simulink model "Hybrid_Series"  (R2017b)
settings: Solver=VariableStepAuto  StartTime=0.0  StopTime=20  RelTol=1e-3  AbsTol=1e-3  EnableMultiTasking=on
model workspace (MATLAB code in the model file):
  | v0                 = 15; % Initial vehicle speed
  | wheel_radius = 0.3; % Wheel radius
  | k                   = 1e-2; % Motor losses (W/(N*M)^2)
  | t_torque        = 0.02; % Electric motor time constant
  | rpm0             = 2000; % Engine initial speed demand
values from neighbouring files (symbols this model uses):
  HEV_Param =     [DataWorkSpace.mat]
libraries: fl_lib x83, nesl_utility x27, sdl_lib x5, elec_lib x2
(part 2 of 2)

== system Hybrid_Series/DC Converter/Thermal Model ==
  Air Temperature : fl_lib/Physical Signals/Sources/PS Constant  constant=HEV_Param.DCDCConv.Air_Temperature
  Ideal Heat Flow Source : fl_lib/Thermal/Thermal Sources/Controlled Heat Flow Rate Source
      settings: SourceProductName=Simscape
  Ideal Temperature Source : fl_lib/Thermal/Thermal Sources/Controlled Temperature Source
      settings: SourceProductName=Simscape
  Nominal Case-Atmosphere Convective Heat Transfer : fl_lib/Thermal/Thermal Elements/Convective Heat Transfer  area=HEV_Param.DCDCConv.Convection.Area cm^2  heat_tr_coeff=HEV_Param.DCDCConv.Convection.HT_Coefficient W/(m^2 *K)  T_specify=off  T_priority=High  T=0 K  T_nominal_specify=off  T_nominal_unit=K  T_nominal_value=1  Q_specify=off  Q_priority=High  Q=0 J/s  Q_nominal_specify=off  Q_nominal_unit=J/s  Q_nominal_value=1
  PtoHeat : fl_lib/Physical Signals/Functions/PS Gain  gain=HEV_Param.DCDCConv.EPower2Heat
  Subsystem : Subsystem
      mask Display: disp('S');
  Temperature Sensor : Subsystem
      mask Display:
      | patch([294.730220921338;294.546109275896;293.995547435362;293.083837611228;291.819760067491;290.215488561913;288.286473106077;286.051291173329;283.531468787557;280.75127321581;277.737479261253;274.519111407178;271.127164295357;267.594304230703;263.954554586898;260.242968142701;256.495289504528;252.747610866356;249.036024422158;245.396274778353;241.8634147137;238.471467601878;235.253099747803;232.239305793246;229.459110221499;226.939287835727;224.704105902979;222.775090447143;221.170818941565;219.906741397828;218.995031573694;218.44446973316;218.260358087718;218.44446973316;218.995031573694;219.906741397828;221.170818941565;222.775090447143;224.704105902979;226.939287835727;229.459110221499;232.239305793247;235.253099747803;238.471467601878;241.8634147137;245.396274778353;249.036024422158;252.747610866356;256.495289504528;260.242968142701;263.954554586898;267.594304230703;271.127164295357;274.519111407178;277.737479261253;280.75127321581;283.531468787557;286.051291173329;288.286473106077;290.215488561913;291.819760067491;293.083837611228;293.995547435362;294.546109275896;294.730220921338;294.730220921338], [122.389574535191;118.641895897019;114.930309452821;111.290559809016;107.757699744363;104.365752632541;101.147384778466;98.1335908239095;95.3533952521624;92.8335728663899;90.598390933642;88.6693754778057;87.0651039722279;85.8010264284914;84.8893166043572;84.3387547638233;84.1546431183815;84.3387547638233;84.8893166043572;85.8010264284914;87.0651039722279;88.6693754778058;90.598390933642;92.83357286639;95.3533952521625;98.1335908239095;101.147384778466;104.365752632541;107.757699744363;111.290559809016;114.930309452821;118.641895897019;122.389574535191;126.137253173364;129.848839617561;133.488589261366;137.02144932602;140.413396437841;143.631764291917;146.645558246473;149.42575381822;151.945576203992;154.18075813674;156.109773592576;157.714045098154;158.978122641891;159.889832466025;160.440394306559;160.624505952001;160.440394306559;159.889832466025;158.978122641891;157.714045098154;156.109773592576;154.18075813674;151.945576203992;149.42575381822;146.645558246473;143.631764291917;140.413396437841;137.02144932602;133.488589261366;129.848839617561;126.137253173364;122.389574535191;122.389574535191], [0;0;0])
      | plot([294.730220921338;294.546109275896;293.995547435362;293.083837611228;291.819760067491;290.215488561913;288.286473106077;286.051291173329;283.531468787557;280.75127321581;277.737479261253;274.519111407178;271.127164295357;267.594304230703;263.954554586898;260.242968142701;256.495289504528;252.747610866356;249.036024422158;245.396274778353;241.8634147137;238.471467601878;235.253099747803;232.239305793246;229.459110221499;226.939287835727;224.704105902979;222.775090447143;221.170818941565;219.906741397828;218.995031573694;218.44446973316;218.260358087718;218.44446973316;218.995031573694;219.906741397828;221.170818941565;222.775090447143;224.704105902979;226.939287835727;229.459110221499;232.239305793247;235.253099747803;238.471467601878;241.8634147137;245.396274778353;249.036024422158;252.747610866356;256.495289504528;260.242968142701;263.954554586898;267.594304230703;271.127164295357;274.519111407178;277.737479261253;280.75127321581;283.531468787557;286.051291173329;288.286473106077;290.215488561913;291.819760067491;293.083837611228;293.995547435362;294.546109275896;294.730220921338;294.730220921338], [122.389574535191;118.641895897019;114.930309452821;111.290559809016;107.757699744363;104.365752632541;101.147384778466;98.1335908239095;95.3533952521624;92.8335728663899;90.598390933642;88.6693754778057;87.0651039722279;85.8010264284914;84.8893166043572;84.3387547638233;84.1546431183815;84.3387547638233;84.8893166043572;85.8010264284914;87.0651039722279;88.6693754778058;90.598390933642;92.83357286639;95.3533952521625;98.1335908239095;101.147384778466;104.365752632541;107.757699744363;111.290559809016;114.930309452821;118.641895897019;122.389574535191;126.137253173364;129.848839617561;133.488589261366;137.02144932602;140.413396437841;143.631764291917;146.645558246473;149.42575381822;151.945576203992;154.18075813674;156.109773592576;157.714045098154;158.978122641891;159.889832466025;160.440394306559;160.624505952001;160.440394306559;159.889832466025;158.978122641891;157.714045098154;156.109773592576;154.18075813674;151.945576203992;149.42575381822;146.645558246473;143.631764291917;140.413396437841;137.02144932602;133.488589261366;129.848839617561;126.137253173364;122.389574535191;122.389574535191])
      | plot([243.771309033036;263.613159768283;263.613159768283;243.771309033036;243.771309033036], [438.410416245461;438.410416245461;112.4371541664;112.4371541664;438.410416245461])
      | plot([510.219018906355;0;0;510.219018906355;510.219018906355], [509.274168871343;509.274168871343;0;0;509.274168871343])
      | ;
      | %color('red');
      | %port_label('LConn', 1,'A')
      | %port_label('RConn', 1,'B')
  Thermal Mass : fl_lib/Thermal/Thermal Elements/Thermal Mass  mass=HEV_Param.DCDCConv.Thermal_Mass kg  sp_heat=HEV_Param.DCDCConv.Specific_Heat J/kg/K  T_specify=on  T_priority=High  T=HEV_Param.DCDCConv.Initial_Temperature degC  T_nominal_specify=off  T_nominal_unit=K  T_nominal_value=1  Q_specify=off  Q_priority=High  Q=0 J/s  Q_nominal_specify=off  Q_nominal_unit=J/s  Q_nominal_value=1
  Thermal Reference : fl_lib/Thermal/Thermal Elements/Thermal Reference
  Thermal Reference1 : fl_lib/Thermal/Thermal Elements/Thermal Reference
  P Loss : PMIOPort  Port=1  Side=Left
  connections:
  Thermal Reference1/LConn1 -- Ideal Heat Flow Source/RConn2
  PtoHeat/LConn1 -- Subsystem/RConn1
  Subsystem/LConn1 -- P Loss/RConn1
  Air Temperature/RConn1 -- Ideal Temperature Source/RConn1
  Ideal Temperature Source/RConn2 -- Thermal Reference/LConn1
  PtoHeat/RConn1 -- Ideal Heat Flow Source/RConn1
  Ideal Heat Flow Source/LConn1 -- Thermal Mass/LConn1 -- Nominal Case-Atmosphere Convective Heat Transfer/RConn1 -- Temperature Sensor/LConn1
  Nominal Case-Atmosphere Convective Heat Transfer/LConn1 -- Ideal Temperature Source/LConn1

== system Hybrid_Series/DC Converter/Voltage Sensor ==
  PS-Simulink Converter : nesl_utility/PS-Simulink Converter  PhysicalDomain=network_engine_domain  SubClassName=ps_output  LeftPortType=input  RightPortType=output  PseudoPeriodic=off  Frequencies=[]  Unit=1  AffineConversion=off
  Voltage Sensor In : fl_lib/Electrical/Electrical Sensors/Voltage Sensor
  + : PMIOPort  Port=1  Side=Left
  V : PMIOPort  Port=2  Side=Right
  - : PMIOPort  Port=3  Side=Right
  tag scope: V_in=global
  wires:
  PS-Simulink Converter/1 -> [V_in]
  connections:
  PS-Simulink Converter/LConn1 -- Voltage Sensor In/RConn1 -- V/RConn1
  -/RConn1 -- Voltage Sensor In/RConn2
  +/RConn1 -- Voltage Sensor In/LConn1

== system Hybrid_Series/DC Converter/Voltage Sensor Bus ==
  PS-Simulink Converter : nesl_utility/PS-Simulink Converter  PhysicalDomain=network_engine_domain  SubClassName=ps_output  LeftPortType=input  RightPortType=output  PseudoPeriodic=off  Frequencies=[]  Unit=1  AffineConversion=off
  Voltage Sensor Out : fl_lib/Electrical/Electrical Sensors/Voltage Sensor
  + : PMIOPort  Port=1  Side=Left
  - : PMIOPort  Port=2  Side=Right
  V : PMIOPort  Port=3  Side=Right
  tag scope: V_out=global
  wires:
  PS-Simulink Converter/1 -> [V_out]
  connections:
  -/RConn1 -- Voltage Sensor Out/RConn2
  PS-Simulink Converter/LConn1 -- Voltage Sensor Out/RConn1 -- V/RConn1
  +/RConn1 -- Voltage Sensor Out/LConn1

== system Hybrid_Series/Engine/Engine Management ==
  rpm_dem : Inport
  rpm : Inport  Port=2
  Kp : Gain  Gain=1e-3  SaturateOnIntegerOverflow=on  OutDataTypeStr=Inherit: Same as input  ParamDataTypeStr=Inherit: Same as input
  Sum2 : Sum  Inputs=+-|  SaturateOnIntegerOverflow=on  InputSameDT=on  OutDataTypeStr=Inherit: Same as first input
  "[0,1]" : Saturate  UpperLimit=1  LowerLimit=0
  T : Outport
  wires:
  rpm/1 -> Sum2/2
  rpm_dem/1 -> Sum2/1
  Sum2/1 -> Kp/1
  Kp/1 -> "[0,1]"/1
  "[0,1]"/1 -> T/1

== system Hybrid_Series/Engine/RPM Sensor ==
  Ideal Rotational Motion Sensor : fl_lib/Mechanical/Mechanical Sensors/Ideal Rotational Motion Sensor  offset=0 rad
  MRR : fl_lib/Mechanical/Rotational Elements/Mechanical Rotational Reference
  PS2S : nesl_utility/PS-Simulink Converter  PhysicalDomain=network_engine_domain  SubClassName=ps_output  LeftPortType=input  RightPortType=output  PseudoPeriodic=off  Frequencies=[]  Unit=rpm  AffineConversion=off
  Sensor dynamics : TransferFcn  Denominator=[0.01 1]
  F : PMIOPort  Port=1  Side=Left
  rpm : Outport
  tag scope: engine_rpm=global
  wires:
  PS2S/1 -> Sensor dynamics/1, [engine_rpm]
  Sensor dynamics/1 -> rpm/1
  connections:
  F/RConn1 -- Ideal Rotational Motion Sensor/LConn1
  Ideal Rotational Motion Sensor/RConn2 -- PS2S/LConn1
  MRR/LConn1 -- Ideal Rotational Motion Sensor/RConn1

== system Hybrid_Series/Engine/Sensor Fuel ==
  Integrator : Integrator
  PS2S2 : nesl_utility/PS-Simulink Converter  PhysicalDomain=network_engine_domain  SubClassName=ps_output  LeftPortType=input  RightPortType=output  PseudoPeriodic=off  Frequencies=[]  Unit=g/s  AffineConversion=off
  FC : PMIOPort  Port=1  Side=Left
  tag scope: Fuel=global
  wires:
  PS2S2/1 -> Integrator/1
  Integrator/1 -> [Fuel]
  connections:
  FC/RConn1 -- PS2S2/LConn1

== system Hybrid_Series/Engine/Sensor Power ==
  PS2S1 : nesl_utility/PS-Simulink Converter  PhysicalDomain=network_engine_domain  SubClassName=ps_output  LeftPortType=input  RightPortType=output  PseudoPeriodic=off  Frequencies=[]  Unit=kW  AffineConversion=off
  P : PMIOPort  Port=1  Side=Left
  tag scope: Pm_engine=global
  wires:
  PS2S1/1 -> [Pm_engine]
  connections:
  P/RConn1 -- PS2S1/LConn1

== system Hybrid_Series/Generator/Power Sensor ==
  Current Sensor : fl_lib/Electrical/Electrical Sensors/Current Sensor
  PS Product1 : fl_lib/Physical Signals/Functions/PS Product
      settings: SourceProductName=Simscape
  PS-Simulink Converter4 : nesl_utility/PS-Simulink Converter  PhysicalDomain=network_engine_domain  SubClassName=ps_output  LeftPortType=input  RightPortType=output  PseudoPeriodic=off  Frequencies=[]  Unit=N*m  AffineConversion=off
  To Workspace : ToWorkspace  VariableName=powerGen  SampleTime=-1
      settings: Save2DSignal=2-D array (concatenate along first dimension)
  Voltage Sensor : fl_lib/Electrical/Electrical Sensors/Voltage Sensor
  W to kW : Gain  Gain=1/1000
  + : PMIOPort  Port=1  Side=Left
  ref : PMIOPort  Port=2  Side=Left
  - : PMIOPort  Port=3  Side=Right
  tag scope: Pe_gen=global
  wires:
  W to kW/1 -> To Workspace/1, [Pe_gen]
  PS-Simulink Converter4/1 -> W to kW/1
  connections:
  Current Sensor/RConn1 -- PS Product1/LConn1
  -/RConn1 -- Current Sensor/RConn2 -- Voltage Sensor/LConn1
  Voltage Sensor/RConn1 -- PS Product1/LConn2
  PS-Simulink Converter4/LConn1 -- PS Product1/RConn1
  +/RConn1 -- Current Sensor/LConn1
  ref/RConn1 -- Voltage Sensor/RConn2

== system Hybrid_Series/Generator/RPM Sensor ==
  Mechanical Rotational Reference : fl_lib/Mechanical/Rotational Elements/Mechanical Rotational Reference
  Motion Sensor : fl_lib/Mechanical/Mechanical Sensors/Ideal Rotational Motion Sensor  offset=0 rad
  PS-Simulink Converter 2 : nesl_utility/PS-Simulink Converter  PhysicalDomain=network_engine_domain  SubClassName=ps_output  LeftPortType=input  RightPortType=output  PseudoPeriodic=off  Frequencies=[]  Unit=rpm  AffineConversion=off
  R : PMIOPort  Port=1  Side=Left
  rpm : Outport
  wires:
  PS-Simulink Converter 2/1 -> rpm/1
  connections:
  Motion Sensor/RConn2 -- PS-Simulink Converter 2/LConn1
  Motion Sensor/RConn1 -- Mechanical Rotational Reference/LConn1
  R/RConn1 -- Motion Sensor/LConn1

== system Hybrid_Series/Generator/Torque Lag ==
  0.2 second lag : fl_lib/Physical Signals/Functions/PS Gain  gain=1/t_torque
  PS Integrator : fl_lib/Physical Signals/Linear Operators/PS Integrator  x0=0
      settings: SourceProductName=Simscape  SourceProductBaseCode=SS
  PS Subtract : fl_lib/Physical Signals/Functions/PS Subtract
      settings: SourceProductName=Simscape
  i : PMIOPort  Port=1  Side=Left
  o : PMIOPort  Port=2  Side=Right
  connections:
  i/RConn1 -- PS Subtract/LConn1
  PS Subtract/LConn2 -- o/RConn1 -- PS Integrator/RConn1
  0.2 second lag/RConn1 -- PS Integrator/LConn1
  PS Subtract/RConn1 -- 0.2 second lag/LConn1

== system Hybrid_Series/Motor/Power Sensor ==
  Current Sensor : fl_lib/Electrical/Electrical Sensors/Current Sensor
  PS Product1 : fl_lib/Physical Signals/Functions/PS Product
      settings: SourceProductName=Simscape
  PS-Simulink Converter4 : nesl_utility/PS-Simulink Converter  PhysicalDomain=network_engine_domain  SubClassName=ps_output  LeftPortType=input  RightPortType=output  PseudoPeriodic=off  Frequencies=[]  Unit=N*m  AffineConversion=off
  To Workspace : ToWorkspace  VariableName=powerMo  SampleTime=-1
      settings: Save2DSignal=2-D array (concatenate along first dimension)
  Voltage Sensor : fl_lib/Electrical/Electrical Sensors/Voltage Sensor
  W to kW : Gain  Gain=1/1000
  + : PMIOPort  Port=1  Side=Left
  ref : PMIOPort  Port=2  Side=Left
  - : PMIOPort  Port=3  Side=Right
  tag scope: Pe_Mo=global
  wires:
  W to kW/1 -> To Workspace/1, [Pe_Mo]
  PS-Simulink Converter4/1 -> W to kW/1
  connections:
  Current Sensor/RConn1 -- PS Product1/LConn1
  -/RConn1 -- Current Sensor/RConn2 -- Voltage Sensor/LConn1
  Voltage Sensor/RConn1 -- PS Product1/LConn2
  PS-Simulink Converter4/LConn1 -- PS Product1/RConn1
  +/RConn1 -- Current Sensor/LConn1
  ref/RConn1 -- Voltage Sensor/RConn2

== system Hybrid_Series/Motor/RPM Sensor ==
  Mechanical Rotational Reference : fl_lib/Mechanical/Rotational Elements/Mechanical Rotational Reference
  Motion Sensor : fl_lib/Mechanical/Mechanical Sensors/Ideal Rotational Motion Sensor  offset=0 rad
  PS-Simulink Converter 2 : nesl_utility/PS-Simulink Converter  PhysicalDomain=network_engine_domain  SubClassName=ps_output  LeftPortType=input  RightPortType=output  PseudoPeriodic=off  Frequencies=[]  Unit=rpm  AffineConversion=off
  R : PMIOPort  Port=1  Side=Left
  rpm : Outport
  wires:
  PS-Simulink Converter 2/1 -> rpm/1
  connections:
  Motion Sensor/RConn2 -- PS-Simulink Converter 2/LConn1
  Motion Sensor/RConn1 -- Mechanical Rotational Reference/LConn1
  R/RConn1 -- Motion Sensor/LConn1

== system Hybrid_Series/Motor/Speed Controller ==
  rpm_ref : Inport
  rpm : Inport  Port=2
  20Hz Lowpass Filter : TransferFcn  Denominator=[1/(2*pi*20) 1]
  Ki : Gain  Gain=60
  Kp : Gain  Gain=60
  Limits [-40,40] : Integrator  LimitOutput=on  UpperSaturationLimit=40  LowerSaturationLimit=-40
  Sum : Sum  Inputs=-+|
  Sum1 : Sum  Inputs=++|
  "[-40,40]" : Saturate  UpperLimit=400  LowerLimit=-400
  T_ref : Outport
  wires:
  rpm_ref/1 -> Sum/2
  rpm/1 -> 20Hz Lowpass Filter/1
  Sum1/1 -> "[-40,40]"/1
  Sum/1 -> Ki/1, Kp/1
  Ki/1 -> Limits [-40,40]/1
  Kp/1 -> Sum1/2
  Limits [-40,40]/1 -> Sum1/1
  20Hz Lowpass Filter/1 -> Sum/1
  "[-40,40]"/1 -> T_ref/1

== system Hybrid_Series/Motor/Torque Lag ==
  0.2 second lag : fl_lib/Physical Signals/Functions/PS Gain  gain=1/t_torque
  PS Integrator : fl_lib/Physical Signals/Linear Operators/PS Integrator  x0=0
      settings: SourceProductName=Simscape  SourceProductBaseCode=SS
  PS Subtract : fl_lib/Physical Signals/Functions/PS Subtract
      settings: SourceProductName=Simscape
  i : PMIOPort  Port=1  Side=Left
  o : PMIOPort  Port=2  Side=Right
  connections:
  i/RConn1 -- PS Subtract/LConn1
  PS Subtract/LConn2 -- o/RConn1 -- PS Integrator/RConn1
  0.2 second lag/RConn1 -- PS Integrator/LConn1
  PS Subtract/RConn1 -- 0.2 second lag/LConn1

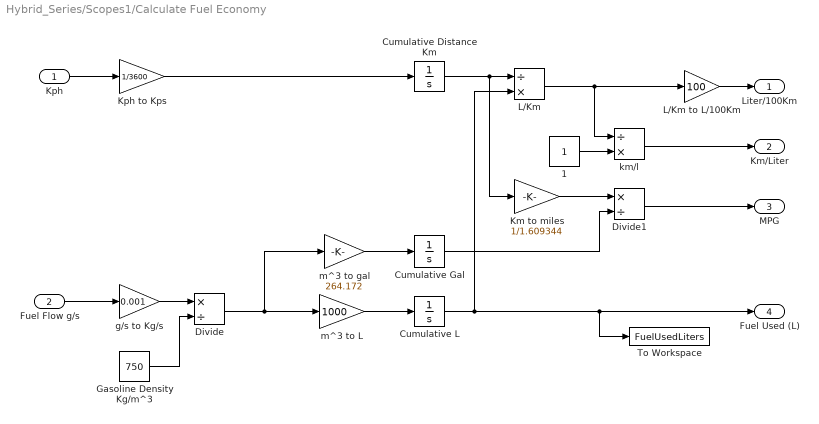
== system Hybrid_Series/Scopes1/Calculate Fuel Economy ==
  Kph : Inport
  Fuel Flow g/s : Inport  Port=2
  1 : Constant
  Cumulative Distance Km : Integrator  InitialCondition=eps
  Cumulative Gal : Integrator  InitialCondition=eps
  Cumulative L : Integrator  InitialCondition=eps
  Divide : Product  Inputs=*/
  Divide1 : Product  Inputs=*/
  Gasoline Density Kg/m^3 : Constant  Value=750
  Km to miles : Gain  Gain=1/1.609344
  Kph to Kps : Gain  Gain=1/3600
  L/Km : Product  Inputs=/*
  L/Km to L/100Km : Gain  Gain=100
  To Workspace : ToWorkspace  VariableName=FuelUsedLiters  SampleTime=-1
      settings: MaxDataPoints=1
  g/s to Kg/s : Gain  Gain=0.001
  km/l : Product  Inputs=/*
  m^3 to L : Gain  Gain=1000
  m^3 to gal : Gain  Gain=264.172
  Liter/100Km : Outport
  Km/Liter : Outport  Port=2
  MPG : Outport  Port=3
  Fuel Used (L) : Outport  Port=4
  wires:
  km/l/1 -> Km/Liter/1
  1/1 -> km/l/2
  Divide1/1 -> MPG/1
  L/Km to L/100Km/1 -> Liter/100Km/1
  Fuel Flow g/s/1 -> g/s to Kg/s/1
  Kph/1 -> Kph to Kps/1
  Cumulative Gal/1 -> Divide1/2
  Km to miles/1 -> Divide1/1
  L/Km/1 -> km/l/1, L/Km to L/100Km/1
  Cumulative Distance Km/1 -> Km to miles/1, L/Km/1
  Cumulative L/1 -> L/Km/2, Fuel Used (L)/1, To Workspace/1
  Kph to Kps/1 -> Cumulative Distance Km/1
  m^3 to gal/1 -> Cumulative Gal/1
  m^3 to L/1 -> Cumulative L/1
  Divide/1 -> m^3 to gal/1, m^3 to L/1
  Gasoline Density Kg/m^3/1 -> Divide/2
  g/s to Kg/s/1 -> Divide/1

== system Hybrid_Series/Vehicle Body/Sensor Speed and Power ==
  Ideal Rotational Motion Sensor : fl_lib/Mechanical/Mechanical Sensors/Ideal Rotational Motion Sensor  offset=0 rad
  Ideal Torque Sensor : fl_lib/Mechanical/Mechanical Sensors/Ideal Torque Sensor
  Mechanical Rotational Reference : fl_lib/Mechanical/Rotational Elements/Mechanical Rotational Reference
  PS-Simulink Converter : nesl_utility/PS-Simulink Converter  PhysicalDomain=network_engine_domain  SubClassName=ps_output  LeftPortType=input  RightPortType=output  PseudoPeriodic=off  Frequencies=[]  Unit=N*m  AffineConversion=off
  PS-Simulink Converter1 : nesl_utility/PS-Simulink Converter  PhysicalDomain=network_engine_domain  SubClassName=ps_output  LeftPortType=input  RightPortType=output  PseudoPeriodic=off  Frequencies=[]  Unit=rad/s  AffineConversion=off
  Product : Product  RndMeth=Zero
  W2kW : Gain  Gain=0.001
  B : PMIOPort  Port=1  Side=Left
  F : PMIOPort  Port=2  Side=Right
  tag scope: Pm_vehicle=global
  wires:
  W2kW/1 -> [Pm_vehicle]
  Product/1 -> W2kW/1
  PS-Simulink Converter/1 -> Product/1
  PS-Simulink Converter1/1 -> Product/2
  connections:
  Mechanical Rotational Reference/LConn1 -- Ideal Rotational Motion Sensor/RConn1
  Ideal Rotational Motion Sensor/LConn1 -- F/RConn1 -- Ideal Torque Sensor/RConn1
  B/RConn1 -- Ideal Torque Sensor/LConn1
  PS-Simulink Converter/LConn1 -- Ideal Torque Sensor/RConn2
  PS-Simulink Converter1/LConn1 -- Ideal Rotational Motion Sensor/RConn2

== system Hybrid_Series/DC Converter/Thermal Model/Subsystem ==
  PS-Simulink Converter1 : nesl_utility/PS-Simulink Converter  PhysicalDomain=network_engine_domain  SubClassName=ps_output  LeftPortType=input  RightPortType=output  PseudoPeriodic=off  Frequencies=[]  Unit=degC  AffineConversion=on
  In : PMIOPort  Port=1  Side=Left
  Out : PMIOPort  Port=2  Side=Right
  tag scope: DCDC_Power_Loss=global
  wires:
  PS-Simulink Converter1/1 -> [DCDC_Power_Loss]
  connections:
  Out/RConn1 -- PS-Simulink Converter1/LConn1 -- In/RConn1

== system Hybrid_Series/DC Converter/Thermal Model/Temperature Sensor ==
  Ideal Temperature Sensor : fl_lib/Thermal/Thermal Sensors/Temperature Sensor
  PS-Simulink Converter : nesl_utility/PS-Simulink Converter  PhysicalDomain=network_engine_domain  SubClassName=ps_output  LeftPortType=input  RightPortType=output  PseudoPeriodic=off  Frequencies=[]  Unit=degC  AffineConversion=on
  Thermal Reference : fl_lib/Thermal/Thermal Elements/Thermal Reference
  Conn2 : PMIOPort  Port=1  Side=Left
  tag scope: DCDC_SYS=global
  wires:
  PS-Simulink Converter/1 -> [DCDC_SYS]  "DCDC_Temp"
  connections:
  Conn2/RConn1 -- Ideal Temperature Sensor/LConn1
  Thermal Reference/LConn1 -- Ideal Temperature Sensor/RConn1
  PS-Simulink Converter/LConn1 -- Ideal Temperature Sensor/RConn2
